simulink model "adcs_top"  (R2024b)
settings: Solver=VariableStepAuto  StartTime=0.0  StopTime=30  RelTol=1e-3
settings Model: Creator=natha  LastModifiedBy=natha

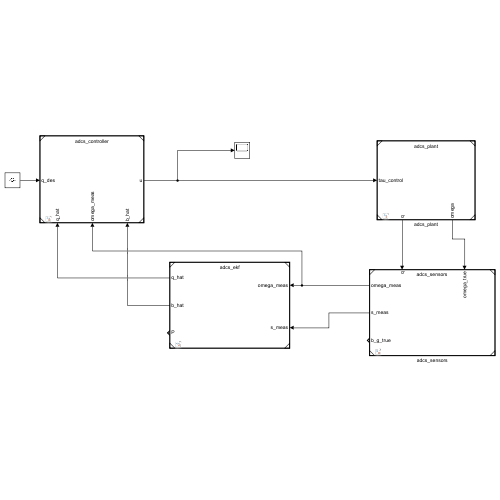
[thumbnail: Simulink's stored preview of the top-level diagram]
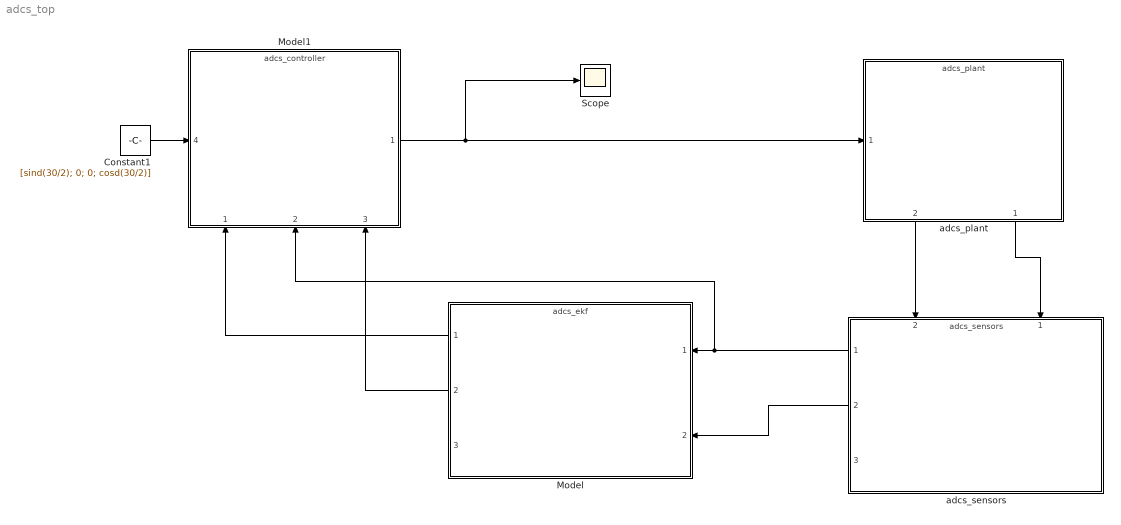
== system adcs_top ==
  Constant1 : Constant  Value=[sind(30/2); 0; 0; cosd(30/2)]
  Model : ModelReference  ModelNameDialog=adcs_ekf  SimulationMode=Normal  ModelReferenceVersion=1.7
      settings: PortSchema="{\"entries\":[{\"content\":{\"sides\":[{\"content\":{\"connectorIds\":[\"Out1\",\"Out2\",\"Out3\"]},\"type\":\"ConnectorPlacement.EquallySpacedRectSide\",\"uuid\":\"e1e8c2f6-347a-40af-a489-4a486dd92b83\"},{\"content\":{\"connectorIds\":[\"In1\",\"In2\"],\"side\":\"RIGHT\"},\"type\":\"ConnectorPlacement.EquallySpacedRectSide\",\"uuid\":\"7d272911-a1f7-467e-adb6-6c23d55756c2\"},{\"content\":{\"side\":\"TOP\"},\"type\":\"ConnectorPlacement.EquallySpacedRectSide\",\"uuid\":\"c6e9175d-15ec-4e70-a8b4-df454a0e0841\"}]},\"type\":\"ConnectorPlacement.EquallySpacedConnector\",\"uuid\":\"e1e20b4a-ad6f-4514-bcaf-182f4cfd2820\"}],\"packageUris\":[\"http://schema.mathworks.com/mf0/Connector/R2020b\"],\"version\":\"1.0\"}"
  Model1 : ModelReference  ModelNameDialog=adcs_controller  SimulationMode=Normal  ModelReferenceVersion=1.3
      settings: PortSchema="{\"entries\":[{\"content\":{\"sides\":[{\"content\":{\"connectorIds\":[\"In4\"]},\"type\":\"ConnectorPlacement.EquallySpacedRectSide\",\"uuid\":\"9a7dce3a-0e24-4f74-8568-077604ed1719\"},{\"content\":{\"connectorIds\":[\"Out1\"],\"side\":\"RIGHT\"},\"type\":\"ConnectorPlacement.EquallySpacedRectSide\",\"uuid\":\"132e05c4-2c3f-48f9-bab4-462e6f54b58f\"},{\"content\":{\"side\":\"TOP\"},\"type\":\"ConnectorPlacement.EquallySpacedRectSide\",\"uuid\":\"948c8154-85c3-48fc-a221-ad950f049ae6\"},{\"content\":{\"connectorIds\":[\"In1\",\"In2\",\"In3\"],\"side\":\"BOTTOM\"},\"type\":\"ConnectorPlacement.EquallySpacedRectSide\",\"uuid\":\"de3e1043-fdca-4441-8ba7-ef689e26219f\"}]},\"type\":\"ConnectorPlacement.EquallySpacedConnector\",\"uuid\":\"d249f73a-2fcc-4096-bae7-3b72d1dc14e2\"}],\"packageUris\":[\"http://schema.mathworks.com/mf0/Connector/R2020b\"],\"version\":\"1.0\"}"
  Scope : Scope
  adcs_plant : ModelReference  ModelNameDialog=adcs_plant  SimulationMode=Normal  ModelReferenceVersion=1.15
      settings: PortSchema="{\"entries\":[{\"content\":{\"sides\":[{\"content\":{\"connectorIds\":[\"In1\"]},\"type\":\"ConnectorPlacement.EquallySpacedRectSide\",\"uuid\":\"eb9888ac-de84-4bc1-a55c-af06666db182\"},{\"content\":{\"side\":\"RIGHT\"},\"type\":\"ConnectorPlacement.EquallySpacedRectSide\",\"uuid\":\"1c97a0d1-5ab9-4f54-a62f-88bfd8ad7da0\"},{\"content\":{\"side\":\"TOP\"},\"type\":\"ConnectorPlacement.EquallySpacedRectSide\",\"uuid\":\"dbf33c93-5dbe-44ed-ac7c-680ab56ff2d7\"},{\"content\":{\"connectorIds\":[\"Out2\",\"Out1\"],\"side\":\"BOTTOM\"},\"type\":\"ConnectorPlacement.EquallySpacedRectSide\",\"uuid\":\"151d038a-e823-469a-a98c-90fa89695792\"}]},\"type\":\"ConnectorPlacement.EquallySpacedConnector\",\"uuid\":\"6876e821-9bc3-492d-80bf-13e76e1de433\"}],\"packageUris\":[\"http://schema.mathworks.com/mf0/Connector/R2020b\"],\"version\":\"1.0\"}"
  adcs_sensors : ModelReference  ModelNameDialog=adcs_sensors  SimulationMode=Normal  ModelReferenceVersion=1.9
      settings: PortSchema="{\"entries\":[{\"content\":{\"sides\":[{\"content\":{\"connectorIds\":[\"Out1\",\"Out2\",\"Out3\"]},\"type\":\"ConnectorPlacement.EquallySpacedRectSide\",\"uuid\":\"e1e8c2f6-347a-40af-a489-4a486dd92b83\"},{\"content\":{\"side\":\"RIGHT\"},\"type\":\"ConnectorPlacement.EquallySpacedRectSide\",\"uuid\":\"7d272911-a1f7-467e-adb6-6c23d55756c2\"},{\"content\":{\"connectorIds\":[\"In2\",\"In1\"],\"side\":\"TOP\"},\"type\":\"ConnectorPlacement.EquallySpacedRectSide\",\"uuid\":\"c6e9175d-15ec-4e70-a8b4-df454a0e0841\"}]},\"type\":\"ConnectorPlacement.EquallySpacedConnector\",\"uuid\":\"e1e20b4a-ad6f-4514-bcaf-182f4cfd2820\"}],\"packageUris\":[\"http://schema.mathworks.com/mf0/Connector/R2020b\"],\"version\":\"1.0\"}"
  wires:
  adcs_plant/1 -> adcs_sensors/1
  adcs_plant/2 -> adcs_sensors/2
  adcs_sensors/2 -> Model/2
  Constant1/1 -> Model1/4
  Model/2 -> Model1/3
  Model/1 -> Model1/1
  Model1/1 -> Scope/1, adcs_plant/1
  adcs_sensors/1 -> Model1/2, Model/1
